simulink model "Ford_T3T6_ArchCnctnDigrm"  (R2016b)
settings: Solver=FixedStepDiscrete  StartTime=0.0  StopTime=10.0  RelTol=1e-3  EnableMultiTasking=on
libraries: canmsglib x15
(part 4 of 15)

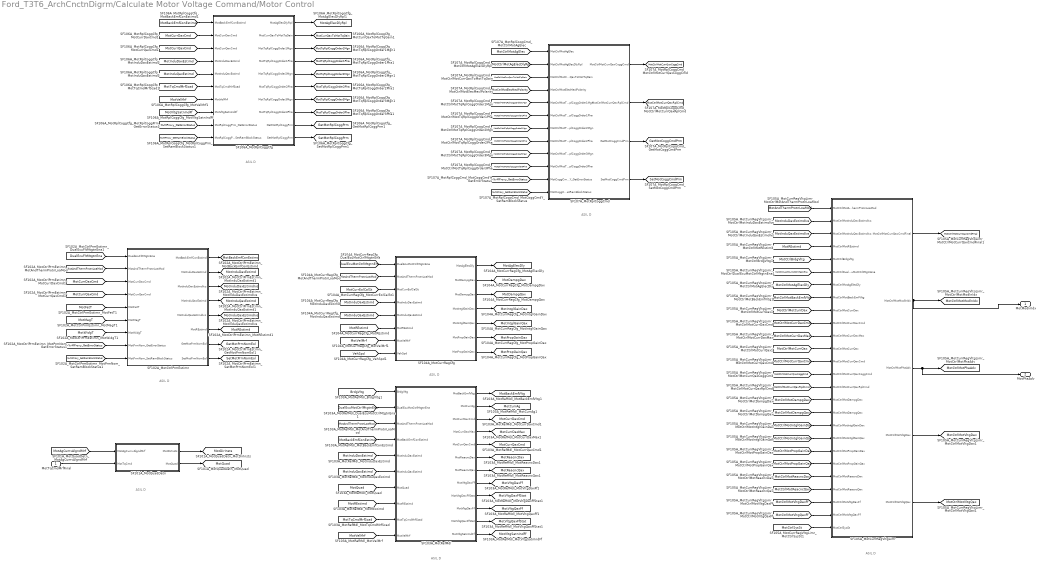
== system Ford_T3T6_ArchCnctnDigrm/Calculate Motor Voltage Command/Motor Control ==
  note: ASIL D
  note: ASIL D
  note: ASIL D
  note: ASIL D
  note: ASIL D
  note: ASIL D
  note: ASIL D
  MotTqCmdMrfFinal : Inport
  SF101A_MotQuadDetn : Subsystem  Tag=1.2.1  Description=The Motor Quadrant Detection function generates an estimate of the motor operating quadrant based on the sign of the Limited Motor Torque Command and the direction of motor shaft motion.
      settings: AttributesFormatString=Version: %<Tag>
  SF102A_MotCtrlPrmEstimn : Subsystem  Tag=3.0.0  Description=The Parameter Compensation function generates four parameter estimates: the Resistance estimate (representing the total motor output circuit resistance), the Ke estimate (representing the motor voltage constant Ke), the q-axis Motor Inductance Estimate and the d-axis Motor Inductance Estimate. The Parameter Compensation function is implemented as a feedforward parameter estimation function based on component nominal values, temperature estimates, the Motor Current Reference (q-axis and d-axis components). The temperature dependent portion of the feedforward parameter estimation function updates synchronously at the same rate as the fastest temperature estimate for the parameter (defined in the Temperature Estimation FDD).
      settings: AttributesFormatString=Version: %<Tag>
  SF103A_MotRefMdl : Subsystem  Tag=4.1.0  Description="The Motor Reference Model Function primary purpose is to calculate the reference motor current in the d/q coordinate frame to be used as the current command for the SF-104A, SF105A Current Regulator.  In general, this calculation produces the optimal (lowest) motor current command reference to produce the Motor Torque Command at the present operating point (motor velocity, supply voltage).  Features are included to use something short of the optimal reference for multiple purposes, such as to reserve some supply voltage budget for downstream current regulator operation, or for cogging/ripple cancellation, or to smooth the transition of low values of Id to high values of Id as the motor operating conditions change.  Supplementary functions include the calculation of a Feedforward Reference Voltage for use in the SF-105A Current Regulator, whose form changes depending on the state of the signal LoA State (this allows operation in Voltage Mode Control in certain fail operational states).  Another supplementary function computes the Motor Reference Current angle (Alpha) for use in the Current Measurement function."
      settings: AttributesFormatString=Version: %<Tag>
  SF104A_MotCurrRegCfg : Subsystem  Tag=3.0.0  Description=The Current Regulator Configuration function generates the following: Proportional and Integral gains for D-axis and Q-axis current regulators, damping terms for D-axis and Q-axis current regulators and a commutation delay compensation value.
      settings: AttributesFormatString=Version: %<Tag>
  SF105A_MotCurrRegVltgLimr : Subsystem  Tag=3.0.0  Description="The Current Regulator and Voltage Limiting function generates the following: Modulation Index, Phase Advance, Final Motor Current Reference Q-axis, Voltage Command D-axis and Voltage Command Q-axis.The Current Regulator portion calculates error signals representing the difference between Motor Reference Currents and Motor Measured Currents, sums in the requested motor current command from the Cogging and Ripple Command Generation function, and uses these corrected error signals modified by proportional and integral gains to generate a portion of the voltage command to the motor.  The Current Regulator also applies separate gains to the measured motor currents to generate an additional portion of the voltage command.  The Feedforward Voltages from the Motor Reference model are added to the other two portions to generate the total requested motor voltage command.The Voltage Limiting portion of the function compares the total requested motor voltage command to the total voltage available at the inverter, and implements a limiting and reference command correcting function in order to prevent windup of Current Regulator states and improve reference command tracking."
      settings: AttributesFormatString=Version: %<Tag>
  SF106A_MotRplCoggCfg : Subsystem  Tag=2.0.0  Description=This function is responsible for computing the magnitude and phase of the torque ripple and cogging torque orders to be cancelled, including base cogging and ripple values and compensation terms for the correcting for the limited bandwidth of the current regulator.
      settings: AttributesFormatString=Version: %<Tag>
  SF107A_MotRplCoggCmd : Subsystem  Tag=1.4.1  Description=This function is responsible for creating the q-axis current command for cogging and torque ripple cancellation.It runs under the time step of MotorControl x2.
      settings: AttributesFormatString=Version: %<Tag>
  MotModlnIdx : Outport
  MotPhaAdv : Outport  Port=2
  tag scope: GetMotCoggCmdPrm=global, GetMotPrmNomEol=global, GetMotRplCoggPrm=global, MotAgElecDly=global, MotAgElecDlyRpl=global, MotBackEmfConEstimd=global, MotBackEmfVltg=global, MotCtrlMotCurrQaxCmdFinal=global, MotCtrlMotCurrQaxCoggCmd=global, MotCtrlMotCurrQaxRplCmd=global, MotCtrlMotModlnIdx=global, MotCtrlMotPhaAdv=global, MotCtrlMotVltgDax=global, MotCtrlMotVltgQax=global, MotCurrAg=global, MotCurrDaxCmd=global, MotCurrDaxMax=global, MotCurrQaxCmd=global, MotCurrQaxToMotTqGain=global, MotDampgDax=global, MotDampgQax=global, MotDirInsts=global, MotInduDaxEstimd=global, MotInduDaxEstimdIvs=global, MotInduQaxEstimd=global, MotInduQaxEstimdIvs=global, MotIntglGainDax=global, MotIntglGainQax=global, MotPropGainDax=global, MotPropGainQax=global, MotQuad=global, MotREstimd=global, MotReacncDax=global, MotReacncQax=global, MotTqRplCoggOrder1Mgn=global, MotTqRplCoggOrder1Pha=global, MotTqRplCoggOrder2Mgn=global, MotTqRplCoggOrder2Pha=global, MotTqRplCoggOrder3Mgn=global, MotTqRplCoggOrder3Pha=global, MotVltgDaxFf=global, MotVltgDaxFfStat=global, MotVltgQaxFf=global, MotVltgQaxFfStat=global, MotVltgSatnIndFf=global, SetMotCoggCmdPrm=global, SetMotPrmNomEol=global, SetMotRplCoggPrm=global
  wires:
  [MotAgCumvAlgndMrf] -> SF101A_MotQuadDetn/1(MotAgCumvAlgndMrf)
  SF101A_MotQuadDetn/2(MotQuad) -> [MotQuad]
  MotTqCmdMrfFinal/1 -> SF101A_MotQuadDetn/2(MotTqCmd)
  SF101A_MotQuadDetn/1(MotDirInsts) -> [MotDirInsts]
  [MotBackEmfConEstimd] -> SF106A_MotRplCoggCfg/1(MotBackEmfConEstimd)
  [MotCurrDaxCmd] -> SF106A_MotRplCoggCfg/2(MotCurrDaxCmd)
  [MotCurrQaxCmd] -> SF106A_MotRplCoggCfg/3(MotCurrQaxCmd)
  [MotInduDaxEstimd] -> SF106A_MotRplCoggCfg/4(MotInduDaxEstimd)
  [MotInduQaxEstimd] -> SF106A_MotRplCoggCfg/5(MotInduQaxEstimd)
  [MotTqCmdMrfScad] -> SF106A_MotRplCoggCfg/6(MotTqCmdMrfScad)
  [MotVelMrf] -> SF106A_MotRplCoggCfg/7(MotVelMrf)
  [MotVltgSatnIndFf] -> SF106A_MotRplCoggCfg/8(MotVltgSatnIndFf)
  [NvMProxy_GetErrorStatus] -> SF106A_MotRplCoggCfg/9(MotRplCoggPrm_GetErrorStatus)
  [NvMProxy_SetRamBlockStatus] -> SF106A_MotRplCoggCfg/10(MotRplCoggPrm_SetRamBlockStatus)
  SF106A_MotRplCoggCfg/1(MotAgElecDlyRpl) -> [MotAgElecDlyRpl]
  SF106A_MotRplCoggCfg/2(MotCurrQaxToMotTqGain) -> [MotCurrQaxToMotTqGain]
  SF106A_MotRplCoggCfg/3(MotTqRplCoggOrder1Mgn) -> [MotTqRplCoggOrder1Mgn]
  SF106A_MotRplCoggCfg/4(MotTqRplCoggOrder1Pha) -> [MotTqRplCoggOrder1Pha]
  SF106A_MotRplCoggCfg/5(MotTqRplCoggOrder2Mgn) -> [MotTqRplCoggOrder2Mgn]
  SF106A_MotRplCoggCfg/6(MotTqRplCoggOrder2Pha) -> [MotTqRplCoggOrder2Pha]
  SF106A_MotRplCoggCfg/7(MotTqRplCoggOrder3Mgn) -> [MotTqRplCoggOrder3Mgn]
  SF106A_MotRplCoggCfg/8(MotTqRplCoggOrder3Pha) -> [MotTqRplCoggOrder3Pha]
  SF106A_MotRplCoggCfg/9(GetMotRplCoggPrm) -> [GetMotRplCoggPrm]
  SF106A_MotRplCoggCfg/10(SetMotRplCoggPrm) -> [SetMotRplCoggPrm]
  [MotAndThermProtnLoaMod] -> SF105A_MotCurrRegVltgLimr/1(MotCtrlMotAndThermProtnLoaMod)
  [MotInduDaxEstimdIvs] -> SF105A_MotCurrRegVltgLimr/2(MotCtrlMotInduDaxEstimdIvs)
  [MotInduQaxEstimdIvs] -> SF105A_MotCurrRegVltgLimr/3(MotCtrlMotInduQaxEstimdIvs)
  [MotREstimd] -> SF105A_MotCurrRegVltgLimr/4(MotCtrlMotREstimd)
  [MotCtrlBrdgVltg] -> SF105A_MotCurrRegVltgLimr/5(MotCtrlBrdgVltg)
  [MotCtrlDualEcuMotCtrlMtgtnEna] -> SF105A_MotCurrRegVltgLimr/6(MotCtrlDualEcuMotCtrlMtgtnEna)
  [MotCtrlMotAgElecDly] -> SF105A_MotCurrRegVltgLimr/7(MotCtrlMotAgElecDly)
  [MotCtrlMotBackEmfVltg] -> SF105A_MotCurrRegVltgLimr/8(MotCtrlMotBackEmfVltg)
  [MotCtrlMotCurrDax] -> SF105A_MotCurrRegVltgLimr/9(MotCtrlMotCurrDax)
  [MotCtrlMotCurrDaxCmd] -> SF105A_MotCurrRegVltgLimr/10(MotCtrlMotCurrDaxCmd)
  [MotCtrlMotCurrDaxMax] -> SF105A_MotCurrRegVltgLimr/11(MotCtrlMotCurrDaxMax)
  [MotCtrlMotCurrQax] -> SF105A_MotCurrRegVltgLimr/12(MotCtrlMotCurrQax)
  [MotCtrlMotCurrQaxCmd] -> SF105A_MotCurrRegVltgLimr/13(MotCtrlMotCurrQaxCmd)
  [MotCtrlMotCurrQaxCoggCmd] -> SF105A_MotCurrRegVltgLimr/14(MotCtrlMotCurrQaxCoggCmd)
  [MotCtrlMotCurrQaxRplCmd] -> SF105A_MotCurrRegVltgLimr/15(MotCtrlMotCurrQaxRplCmd)
  [MotCtrlMotDampgDax] -> SF105A_MotCurrRegVltgLimr/16(MotCtrlMotDampgDax)
  [MotCtrlMotDampgQax] -> SF105A_MotCurrRegVltgLimr/17(MotCtrlMotDampgQax)
  [MotCtrlMotIntglGainDax] -> SF105A_MotCurrRegVltgLimr/18(MotCtrlMotIntglGainDax)
  [MotCtrlMotIntglGainQax] -> SF105A_MotCurrRegVltgLimr/19(MotCtrlMotIntglGainQax)
  [MotCtrlMotPropGainDax] -> SF105A_MotCurrRegVltgLimr/20(MotCtrlMotPropGainDax)
  [MotCtrlMotPropGainQax] -> SF105A_MotCurrRegVltgLimr/21(MotCtrlMotPropGainQax)
  [MotCtrlMotReacncDax] -> SF105A_MotCurrRegVltgLimr/22(MotCtrlMotReacncDax)
  [MotCtrlMotReacncQax] -> SF105A_MotCurrRegVltgLimr/23(MotCtrlMotReacncQax)
  [MotCtrlMotVltgDaxFf] -> SF105A_MotCurrRegVltgLimr/24(MotCtrlMotVltgDaxFf)
  [MotCtrlMotVltgQaxFf] -> SF105A_MotCurrRegVltgLimr/25(MotCtrlMotVltgQaxFf)
  [MotCtrlSysSt] -> SF105A_MotCurrRegVltgLimr/26(MotCtrlSysSt)
  SF105A_MotCurrRegVltgLimr/1(MotCtrlMotCurrQaxCmdFinal) -> [MotCtrlMotCurrQaxCmdFinal]
  SF105A_MotCurrRegVltgLimr/2(MotCtrlMotModlnIdx) -> MotModlnIdx/1, [MotCtrlMotModlnIdx]
  SF105A_MotCurrRegVltgLimr/3(MotCtrlMotPhaAdv) -> MotPhaAdv/1, [MotCtrlMotPhaAdv]
  SF105A_MotCurrRegVltgLimr/4(MotCtrlMotVltgDax) -> [MotCtrlMotVltgDax]
  SF105A_MotCurrRegVltgLimr/5(MotCtrlMotVltgQax) -> [MotCtrlMotVltgQax]
  [DualEcuMotCtrlMtgtnEna] -> SF104A_MotCurrRegCfg/1(DualEcuMotCtrlMtgtnEna)
  [MotAndThermProtnLoaMod] -> SF104A_MotCurrRegCfg/2(MotAndThermProtnLoaMod)
  [MotCurrEolCalSt] -> SF104A_MotCurrRegCfg/3(MotCurrEolCalSt)
  [MotInduDaxEstimd] -> SF104A_MotCurrRegCfg/4(MotInduDaxEstimd)
  [MotInduQaxEstimd] -> SF104A_MotCurrRegCfg/5(MotInduQaxEstimd)
  [MotREstimd] -> SF104A_MotCurrRegCfg/6(MotREstimd)
  [MotVelMrf] -> SF104A_MotCurrRegCfg/7(MotVelMrf)
  [VehSpd] -> SF104A_MotCurrRegCfg/8(VehSpd)
  SF104A_MotCurrRegCfg/1(MotAgElecDly) -> [MotAgElecDly]
  SF104A_MotCurrRegCfg/2(MotDampgDax) -> [MotDampgDax]
  SF104A_MotCurrRegCfg/3(MotDampgQax) -> [MotDampgQax]
  SF104A_MotCurrRegCfg/4(MotIntglGainDax) -> [MotIntglGainDax]
  SF104A_MotCurrRegCfg/5(MotIntglGainQax) -> [MotIntglGainQax]
  SF104A_MotCurrRegCfg/6(MotPropGainDax) -> [MotPropGainDax]
  SF104A_MotCurrRegCfg/7(MotPropGainQax) -> [MotPropGainQax]
  [BrdgVltg] -> SF103A_MotRefMdl/1(BrdgVltg)
  [DualEcuMotCtrlMtgtnEna] -> SF103A_MotRefMdl/2(DualEcuMotCtrlMtgtnEna)
  [MotAndThermProtnLoaMod] -> SF103A_MotRefMdl/3(MotAndThermProtnLoaMod)
  [MotBackEmfConEstimd] -> SF103A_MotRefMdl/4(MotBackEmfConEstimd)
  [MotInduDaxEstimd] -> SF103A_MotRefMdl/5(MotInduDaxEstimd)
  [MotInduQaxEstimd] -> SF103A_MotRefMdl/6(MotInduQaxEstimd)
  [MotQuad] -> SF103A_MotRefMdl/7(MotQuad)
  [MotREstimd] -> SF103A_MotRefMdl/8(MotREstimd)
  [MotTqCmdMrfScad] -> SF103A_MotRefMdl/9(MotTqCmdMrfScad)
  [MotVelMrf] -> SF103A_MotRefMdl/10(MotVelMrf)
  SF103A_MotRefMdl/1(MotBackEmfVltg) -> [MotBackEmfVltg]
  SF103A_MotRefMdl/2(MotCurrAg) -> [MotCurrAg]
  SF103A_MotRefMdl/3(MotCurrDaxCmd) -> [MotCurrDaxCmd]
  SF103A_MotRefMdl/4(MotCurrDaxMax) -> [MotCurrDaxMax]
  SF103A_MotRefMdl/5(MotCurrQaxCmd) -> [MotCurrQaxCmd]
  SF103A_MotRefMdl/6(MotReacncDax) -> [MotReacncDax]
  SF103A_MotRefMdl/7(MotReacncQax) -> [MotReacncQax]
  SF103A_MotRefMdl/8(MotVltgDaxFf) -> [MotVltgDaxFf]
  SF103A_MotRefMdl/9(MotVltgDaxFfStat) -> [MotVltgDaxFfStat]
  SF103A_MotRefMdl/10(MotVltgQaxFf) -> [MotVltgQaxFf]
  SF103A_MotRefMdl/11(MotVltgQaxFfStat) -> [MotVltgQaxFfStat]
  SF103A_MotRefMdl/12(MotVltgSatnIndFf) -> [MotVltgSatnIndFf]
  [DualEcuFltMtgtnEna] -> SF102A_MotCtrlPrmEstimn/1(DualEcuFltMtgtnEna)
  [MotAndThermProtnLoaMod] -> SF102A_MotCtrlPrmEstimn/2(MotAndThermProtnLoaMod)
  [MotCurrDaxCmd] -> SF102A_MotCtrlPrmEstimn/3(MotCurrDaxCmd)
  [MotCurrQaxCmd] -> SF102A_MotCtrlPrmEstimn/4(MotCurrQaxCmd)
  [MotFetT] -> SF102A_MotCtrlPrmEstimn/5(MotFetT)
  [MotMagT] -> SF102A_MotCtrlPrmEstimn/6(MotMagT)
  [MotWidgT] -> SF102A_MotCtrlPrmEstimn/7(MotWidgT)
  [NvMProxy_GetErrorStatus] -> SF102A_MotCtrlPrmEstimn/8(MotPrmNom_GetErrorStatus)
  [NvMProxy_SetRamBlockStatus] -> SF102A_MotCtrlPrmEstimn/9(MotPrmNom_SetRamBlockStatus)
  SF102A_MotCtrlPrmEstimn/1(MotBackEmfConEstimd) -> [MotBackEmfConEstimd]
  SF102A_MotCtrlPrmEstimn/2(MotInduDaxEstimd) -> [MotInduDaxEstimd]
  SF102A_MotCtrlPrmEstimn/3(MotInduDaxEstimdIvs) -> [MotInduDaxEstimdIvs]
  SF102A_MotCtrlPrmEstimn/4(MotInduQaxEstimd) -> [MotInduQaxEstimd]
  SF102A_MotCtrlPrmEstimn/5(MotInduQaxEstimdIvs) -> [MotInduQaxEstimdIvs]
  SF102A_MotCtrlPrmEstimn/6(MotREstimd) -> [MotREstimd]
  SF102A_MotCtrlPrmEstimn/7(GetMotPrmNomEol) -> [GetMotPrmNomEol]
  SF102A_MotCtrlPrmEstimn/8(SetMotPrmNomEol) -> [SetMotPrmNomEol]
  [MotCtrlMotAgElec] -> SF107A_MotRplCoggCmd/1(MotCtrlMotAgElec)
  [MotCtrlMotAgElecDlyRpl] -> SF107A_MotRplCoggCmd/2(MotCtrlMotAgElecDlyRpl)
  [MotCtrlMotCurrQaxToMotTqGain] -> SF107A_MotRplCoggCmd/3(MotCtrlMotCurrQaxToMotTqGain)
  [MotCtrlMotElecMeclPolarity] -> SF107A_MotRplCoggCmd/4(MotCtrlMotElecMeclPolarity)
  [MotCtrlMotTqRplCoggOrder1Mgn] -> SF107A_MotRplCoggCmd/5(MotCtrlMotTqRplCoggOrder1Mgn)
  [MotCtrlMotTqRplCoggOrder1Pha] -> SF107A_MotRplCoggCmd/6(MotCtrlMotTqRplCoggOrder1Pha)
  [MotCtrlMotTqRplCoggOrder2Mgn] -> SF107A_MotRplCoggCmd/7(MotCtrlMotTqRplCoggOrder2Mgn)
  [MotCtrlMotTqRplCoggOrder2Pha] -> SF107A_MotRplCoggCmd/8(MotCtrlMotTqRplCoggOrder2Pha)
  [MotCtrlMotTqRplCoggOrder3Mgn] -> SF107A_MotRplCoggCmd/9(MotCtrlMotTqRplCoggOrder3Mgn)
  [MotCtrlMotTqRplCoggOrder3Pha] -> SF107A_MotRplCoggCmd/10(MotCtrlMotTqRplCoggOrder3Pha)
  [NvMProxy_GetErrorStatus] -> SF107A_MotRplCoggCmd/11(MotCoggCmdY_GetErrorStatus)
  [NvMProxy_SetRamBlockStatus] -> SF107A_MotRplCoggCmd/12(MotCoggCmdY_SetRamBlockStatus)
  SF107A_MotRplCoggCmd/1(MotCtrlMotCurrQaxCoggCmd) -> [MotCtrlMotCurrQaxCoggCmd]
  SF107A_MotRplCoggCmd/2(MotCtrlMotCurrQaxRplCmd) -> [MotCtrlMotCurrQaxRplCmd]
  SF107A_MotRplCoggCmd/3(GetMotCoggCmdPrm) -> [GetMotCoggCmdPrm]
  SF107A_MotRplCoggCmd/4(SetMotCoggCmdPrm) -> [SetMotCoggCmdPrm]

== system Ford_T3T6_ArchCnctnDigrm/Calculate Motor Voltage Command/SF019B_PwrLimr ==
  AltFltActv : Inport
  BrdgVltg : Inport  Port=2
  DualEcuFltMtgtnSca : Inport  Port=3
  MotAndThermProtnLoaMod : Inport  Port=4
  MotBackEmfConEstimd : Inport  Port=5
  MotTqCmdMrf : Inport  Port=6
  MotVelMrf : Inport  Port=7
  GetRefTmr100MicroSec32bit : Inport  Port=8
  GetTiSpan100MicroSec32bit : Inport  Port=9
  SetNtcSts : Inport  Port=10
  MotTqCmdPwrLimd : Outport
  PwrLimrRednFac : Outport  Port=2

== system Ford_T3T6_ArchCnctnDigrm/Calculate Motor Voltage Command/SF032A_MotTqCmdSca1 ==
  MotTqCmdMrf : Inport
  MotTqScaFac_GetErrorStatus : Inport  Port=2
  MotTqScaFac_SetRamBlockStatus : Inport  Port=3
  MotTqCmdMrfScad : Outport
  GetMotTqCmdSca : Outport  Port=2
  SetMotTqCmdSca : Outport  Port=3

== system Ford_T3T6_ArchCnctnDigrm/Calculate Motor Voltage Command/SF050A_MotTqTranlDampg ==
  AssiMechPolarity : Inport
  DiagcStsCtrldShtDwnFltPrsnt : Inport  Port=2
  HwAg : Inport  Port=3
  LoaSt : Inport  Port=4
  MotTqCmdCrf : Inport  Port=5
  MotVelCrf : Inport  Port=6
  SysSt : Inport  Port=7
  VehSpd : Inport  Port=8
  GetRefTmr100MicroSec32bit : Inport  Port=9
  GetTiSpan100MicroSec32bit : Inport  Port=10
  MotTqCmdCrfDampd : Outport
  MotTqCmdMrfDampd : Outport  Port=2
  MotTqTranlDampgCmpl : Outport  Port=3

== system Ford_T3T6_ArchCnctnDigrm/Complex Drivers/AR102B_NxtrTi ==
  ClrErrInjReg : Inport
  ReadErrInjReg : Inport  Port=2
  SetNtcSts : Inport  Port=3
  GetRefTmr100MicroSec32bit : Outport
  GetRefTmr1MicroSec32bit : Outport  Port=2
  GetTiSpan100MicroSec32bit : Outport  Port=3
  GetTiSpan1MicroSec32bit : Outport  Port=4

== system Ford_T3T6_ArchCnctnDigrm/Complex Drivers/CM101B_ExcpnHndlg ==
  SetNtcSts : Inport
  SetNtcStsAndSnpshtData : Inport  Port=2
  ChkForStrtUpTest : Outport
  FeNmiBusBrdgErr : Outport  Port=2
  FeNmiBusSngBitEccErr : Outport  Port=3
  FeNmiClkMonr0RtErr : Outport  Port=4
  FeNmiClkMonr1RtErr : Outport  Port=5
  FeNmiClkMonr2RtErr : Outport  Port=6
  FeNmiClkMonr3RtErr : Outport  Port=7
  FeNmiClkMonr5RtErr : Outport  Port=8
  FeNmiCodFlsEccAdrOvfErr : Outport  Port=9
  FeNmiCodFlsIllglAcsBySysBus : Outport  Port=10
  FeNmiDmaIllglAcsErr : Outport  Port=11
  FeNmiDmaLockStepErrOrGblRamWrBufErr : Outport  Port=12
  FeNmiDmaTrfErr : Outport  Port=13
  FeNmiDtsRamDblBitEccErr : Outport  Port=14
  FeNmiEcmMstChkrErr : Outport  Port=15
  FeNmiFlsSeqErr : Outport  Port=16
  FeNmiGblRamIllglAcsByProcr : Outport  Port=17
  FeNmiGblRamIllglAcsBySysBus : Outport  Port=18
  FeNmiGlbRamEccAdrOvfErr : Outport  Port=19
  FeNmiGtmRamDblBitEccErr : Outport  Port=20
  FeNmiLclRamEccAdrOvfErr : Outport  Port=21
  FeNmiModErrDbgActv : Outport  Port=22
  FeNmiModErrProgmModActv : Outport  Port=23
  FeNmiModErrTestModActv : Outport  Port=24
  FeNmiModErrUsrModInactv : Outport  Port=25
  FeNmiPegErr : Outport  Port=26
  FeNmiProcrLockStepErr : Outport  Port=27
  FeNmiPrphlRamEccAdrOvfErr : Outport  Port=28
  FeNmiResdAreaIllglAcsByHiSpdBus : Outport  Port=29
  FeNmiWdgErr : Outport  Port=30
  GetMcuDiagcIdnData : Outport  Port=31
  GetMcuDiagcSpplData : Outport  Port=32
  ProcMpuExcpnErr : Outport  Port=33
  ProcNonCritOsErr : Outport  Port=34
  ProcPrmntOsErr : Outport  Port=35
  ProcPrvlgdInstrExcpnErr : Outport  Port=36
  ProcUkwnExcpnErr : Outport  Port=37
  SetMcuDiagcIdnData : Outport  Port=38

== system Ford_T3T6_ArchCnctnDigrm/Complex Drivers/CM102B_FlsMem ==
  ChkForStrtUpTest : Inport
  GetRefTmr100MicroSec32bit : Inport  Port=2
  GetTiSpan100MicroSec32bit : Inport  Port=3
  ResvCrcHwUnit : Inport  Port=4
  SetNtcSts : Inport  Port=5
  CodFlsCrcChkCmpl : Outport
  SwApplCrc : Outport  Port=2

== system Ford_T3T6_ArchCnctnDigrm/Complex Drivers/CM103B_RamMem ==
  SetNtcSts : Inport
  GlbRamEccSngBitCntrOutp : Outport
  LclRamEccSngBitCntrOutp : Outport  Port=2

== system Ford_T3T6_ArchCnctnDigrm/Complex Drivers/CM104B_EcmOutpAndDiagc ==
  ChkForStrtUpTest : Inport
  GetMcuDiagcIdnData : Inport  Port=2
  SetMcuDiagcIdnData : Inport  Port=3
  CtrlErrOut : Outport

== system Ford_T3T6_ArchCnctnDigrm/Complex Drivers/CM106B_McuCoreCfgAndDiagc ==
  GetMcuDiagcIdnData : Inport
  SetMcuDiagcIdnData : Inport  Port=2

== system Ford_T3T6_ArchCnctnDigrm/Complex Drivers/CM109B_ClkCfgAndMon ==

== system Ford_T3T6_ArchCnctnDigrm/Complex Drivers/CM800A_SyncCrc ==
  Calc16BitCrc_u08 : Outport
  Calc16BitCrc_u16 : Outport  Port=2
  Calc32BitCrc_u08 : Outport  Port=3
  Calc32BitCrc_u16 : Outport  Port=4
  Calc32BitCrc_u32 : Outport  Port=5
  Calc8BitCrc : Outport  Port=6
  Calc8BitCrc0X2F : Outport  Port=7
  ResvCrcHwUnit : Outport  Port=8

== system Ford_T3T6_ArchCnctnDigrm/Complex Drivers/ES104B_XcpIf ==

== system Ford_T3T6_ArchCnctnDigrm/Complex Drivers/Ford001A_ChkPt ==

== system Ford_T3T6_ArchCnctnDigrm/Complex Drivers/Platform Config ==
  note: how to connect to fast loop??
  note: Not Required
      | Using only one HwAg Sensor
  note: Not Required
      | Using only 4 HwTq Sensors
  note: Not Required
      | Using only 3 MotAg Sensors
  note: how to connect to fast loop??
  note: how to connect to fast loop??
  note: ASIL D
  note: ASIL D
  note: ASIL D
  note: ASIL D
  CM107B_GuardCfgAndDiagc : Subsystem  Tag=1.2.0  Description=FDD that contians guard configuration for PEG, IPG, HBG, GRG and PBG
      settings: AttributesFormatString=Version: %<Tag>
  CM201A_DmaCfgAndUse : Subsystem  Tag=1.2.0  Description=DMA Configuration and Usage
      settings: AttributesFormatString=Version: %<Tag>
  CM301A_Adcf0CfgAndUse : Subsystem  Tag=1.1.0  Description="This FDD is responsible for configuring and use of the Adcf0.  This is the Adc sampled at the motor control rate."
      settings: AttributesFormatString=Version: %<Tag>
  CM321A_Adcf1CfgAndUse : Subsystem  Tag=1.1.0  Description="This FDD is responsible for configuring and use of the ADC1.  This is the ADC sampled at the 2mSec rate."
      settings: AttributesFormatString=Version: %<Tag>
  ES102A_PolarityCfg : Subsystem  Tag=1.4.0  Description=Identifies polarity control settings for certain points in the design
      settings: AttributesFormatString=Version: %<Tag>
  tag scope: Adcf1EnaCnvn=global, AssiMechPolarity=global, DmaEna2MilliSecToMotCtrlTrf=global, DmaWaitForMotCtrlTo2MilliSecTrf=global, HwAgAPolarity=global, HwAgBPolarity=global, HwAgCPolarity=global, HwAgDPolarity=global, HwAgEPolarity=global, HwAgFPolarity=global, HwAgGPolarity=global, HwAgHPolarity=global, HwTqAPolarity=global, HwTqBPolarity=global, HwTqCPolarity=global, HwTqDPolarity=global, HwTqEPolarity=global, HwTqFPolarity=global, HwTqGPolarity=global, HwTqHPolarity=global, InjDmaErr=global, InjMcuDiagcErr=global, MotAgMeclAPolarity=global, MotAgMeclBPolarity=global, MotAgMeclCPolarity=global, MotAgMeclDPolarity=global, MotAgMeclEPolarity=global, MotAgMeclFPolarity=global, MotAgMeclGPolarity=global, MotAgMeclHPolarity=global, MotCtrlAdc0RawRes=global, MotCtrlAdc1RawRes=global, MotCtrlMgr_MotCtrlFromTwoMilliSec_Rec=global, MotCtrlMgr_TwoMilliSecFromMotCtrl_Rec=global, MotElecMeclPolarity=global, PolarityCfgRead=global, PolarityCfgWr=global
  wires:
  [MotCtrlAdcDiagcEndPtrOutp] -> CM301A_Adcf0CfgAndUse/1(MotCtrlAdcDiagcEndPtrOutp)
  [MotCtrlAdcDiagcStrtPtrOutp] -> CM301A_Adcf0CfgAndUse/2(MotCtrlAdcDiagcStrtPtrOutp)
  [AdcDiagcEndPtrOutp] -> CM321A_Adcf1CfgAndUse/1(AdcDiagcEndPtrOutp)
  [AdcDiagcStrtPtrOutp] -> CM321A_Adcf1CfgAndUse/2(AdcDiagcStrtPtrOutp)
  CM321A_Adcf1CfgAndUse/1(Adcf1EnaCnvn) -> [Adcf1EnaCnvn]
  [MotCtrlMgr_MotCtrlToTwoMilliSec_Rec] -> CM201A_DmaCfgAndUse/1(MotCtrlMgr_MotCtrlToTwoMilliSec_Rec)
  [MotCtrlMgr_TwoMilliSecToMotCtrl_Rec] -> CM201A_DmaCfgAndUse/2(MotCtrlMgr_TwoMilliSecToMotCtrl_Rec)
  [Adc1CfgAndUseAdc1EnaCnvn] -> CM201A_DmaCfgAndUse/3(Adc1CfgAndUseAdc1EnaCnvn)
  [ClrErrInjReg] -> CM201A_DmaCfgAndUse/4(ClrErrInjReg)
  [GetRefTmr1MicroSec32bit] -> CM201A_DmaCfgAndUse/5(GetRefTmr1MicroSec32bit)
  [GetTiSpan1MicroSec32bit] -> CM201A_DmaCfgAndUse/6(GetTiSpan1MicroSec32bit)
  [ReadErrInjReg] -> CM201A_DmaCfgAndUse/7(ReadErrInjReg)
  [StrtErrInjCntr] -> CM201A_DmaCfgAndUse/8(StrtErrInjCntr)
  CM201A_DmaCfgAndUse/1(MotCtrlAdc0RawRes) -> [MotCtrlAdc0RawRes]
  CM201A_DmaCfgAndUse/2(MotCtrlAdc1RawRes) -> [MotCtrlAdc1RawRes]
  CM201A_DmaCfgAndUse/3(MotCtrlMgr_MotCtrlFromTwoMilliSec_Rec) -> [MotCtrlMgr_MotCtrlFromTwoMilliSec_Rec]
  CM201A_DmaCfgAndUse/4(MotCtrlMgr_TwoMilliSecFromMotCtrl_Rec) -> [MotCtrlMgr_TwoMilliSecFromMotCtrl_Rec]
  CM201A_DmaCfgAndUse/5(DmaEna2MilliSecToMotCtrlTrf) -> [DmaEna2MilliSecToMotCtrlTrf]
  CM201A_DmaCfgAndUse/6(DmaWaitForMotCtrlTo2MilliSecTrf) -> [DmaWaitForMotCtrlTo2MilliSecTrf]
  CM201A_DmaCfgAndUse/7(InjDmaErr) -> [InjDmaErr]
  CM201A_DmaCfgAndUse/8(InjMcuDiagcErr) -> [InjMcuDiagcErr]
  [NvMProxy_SetRamBlockStatus] -> ES102A_PolarityCfg/1(PolarityCfgSaved_SetRamBlockStatus)
  ES102A_PolarityCfg/1(AssiMechPolarity) -> [AssiMechPolarity]
  ES102A_PolarityCfg/2(HwAgAPolarity) -> [HwAgAPolarity]
  ES102A_PolarityCfg/3(HwAgBPolarity) -> [HwAgBPolarity]
  ES102A_PolarityCfg/4(HwAgCPolarity) -> [HwAgCPolarity]
  ES102A_PolarityCfg/5(HwAgDPolarity) -> [HwAgDPolarity]
  ES102A_PolarityCfg/6(HwAgEPolarity) -> [HwAgEPolarity]
  ES102A_PolarityCfg/7(HwAgFPolarity) -> [HwAgFPolarity]
  ES102A_PolarityCfg/8(HwAgGPolarity) -> [HwAgGPolarity]
  ES102A_PolarityCfg/9(HwAgHPolarity) -> [HwAgHPolarity]
  ES102A_PolarityCfg/10(HwTqAPolarity) -> [HwTqAPolarity]
  ES102A_PolarityCfg/11(HwTqBPolarity) -> [HwTqBPolarity]
  ES102A_PolarityCfg/12(HwTqCPolarity) -> [HwTqCPolarity]
  ES102A_PolarityCfg/13(HwTqDPolarity) -> [HwTqDPolarity]
  ES102A_PolarityCfg/14(HwTqEPolarity) -> [HwTqEPolarity]
  ES102A_PolarityCfg/15(HwTqFPolarity) -> [HwTqFPolarity]
  ES102A_PolarityCfg/16(HwTqGPolarity) -> [HwTqGPolarity]
  ES102A_PolarityCfg/17(HwTqHPolarity) -> [HwTqHPolarity]
  ES102A_PolarityCfg/18(MotAgMeclAPolarity) -> [MotAgMeclAPolarity]
  ES102A_PolarityCfg/19(MotAgMeclBPolarity) -> [MotAgMeclBPolarity]
  ES102A_PolarityCfg/20(MotAgMeclCPolarity) -> [MotAgMeclCPolarity]
  ES102A_PolarityCfg/21(MotAgMeclDPolarity) -> [MotAgMeclDPolarity]
  ES102A_PolarityCfg/22(MotAgMeclEPolarity) -> [MotAgMeclEPolarity]
  ES102A_PolarityCfg/23(MotAgMeclFPolarity) -> [MotAgMeclFPolarity]
  ES102A_PolarityCfg/24(MotAgMeclGPolarity) -> [MotAgMeclGPolarity]
  ES102A_PolarityCfg/25(MotAgMeclHPolarity) -> [MotAgMeclHPolarity]
  ES102A_PolarityCfg/26(MotElecMeclPolarity) -> [MotElecMeclPolarity]
  ES102A_PolarityCfg/27(PolarityCfgRead) -> [PolarityCfgRead]
  ES102A_PolarityCfg/28(PolarityCfgWr) -> [PolarityCfgWr]

== system Ford_T3T6_ArchCnctnDigrm/Development/DF001A_FltInj ==
  HwVel : Inport
  GetRefTmr100MicroSec32bit : Inport  Port=2
  GetTiSpan100MicroSec32bit : Inport  Port=3
  FltInj_f32 : Outport
  FltInj_logl : Outport  Port=2
  FltInj_u08 : Outport  Port=3
  FltInj_u0p16 : Outport  Port=4

== system Ford_T3T6_ArchCnctnDigrm/Ford CFs/Customer Diag Services ==
  note: EED0
  note: DE00
  note: 3F964_REQ_05050300v2: SES
      | End of Travel Learning
      |
      | SES_Enabled (Software End Stops) Boolean
      | SESCompensatedSPA
      | EndStopsLearned
      | MaxAngleTavel
      | SESRampDownRate
      | SESDampUpRate
  note: EAC: External Angle Command: Kind of automated steering
  note: ANC_Enabled
      | No Units
      | Bool
      |
      | PDC_Enabled
      | No Units
      | Bool
      |
      | TSC_Enabled
      | No Units
      | Bool
      |
      | BPR_Enabled
      | No Units
      | Bool
      |
      | LKA_Enabled
      | No Units
      | Bool
      |
      | LDW_Enabled
      | No Units
      | Bool
      |
      | TJA_Enabled
      | No Units
      | Bool
      |
      | LCA_Enabled
      | No Units
      | Bool
      |
      | TBA_Enabled
      | No Units
      | Bool
      |
      | TBA_5_Wheel_Enabled
      | No Units
      | Bool
      |
      | TBA_TRG_Enabled
      | No Units
      | Bool
      |
      | ESA_Enabled
      | No Units
      | Bool
      |
      | DSR_Enabled
      | No Units
      | Bool
      |
      | SAPP/APA_Enabled
      | No Units
      | Bool
      |
      | SES_Enabled
      | No Units
      | Bool
      |
      | StartStop_Enabled (StrtStopDIDSt)
      | No Units
      | U-8
      |
      | ActiveReturn_Enabled
      | No Units
      | Bool
      |
      | SDM_Enabled
      | No Units
      | Bool
      |
      | RF_Enabled
      | No Units
      | Bool
      |
      | AFS_Present
      | No Units
      | Bool
  note: DE00 Byte 5
  note: DE02 Byte 1
  note: DE01 Byte 1
  note: DE00 Byte 4
  note: DE01 Byte 2
  note: DE01 Byte 3
  note: DE01 Byte 4 ??
  note: DE02 Byte 4 ??
  note: DE01 Byte 5
  note: DE01 Byte 6
  note: DE01 Byte 7
  note: DE01 Byte 8
  note: DE01 Byte 9
  note: DE01 Byte 9
  note: DE01 Byte 9
  note: DE01 Byte 10
  note: DE01 Byte 23
  note: DE02 Byte 5
  note: DE02 Byte 6
  note: DE01 Byte 5
  note: DE01
  note: DE02
  note: DE03
  note: EE00
  note: EE01
  note: EE02
  note: EE20
  note: EE21
  note: EE22
  note: EE23
  note: EE40
  note: EE41
  note: EE42
  note: EE43
  note: EE80
  note: EED1
  note: EED2
  CF086_FordDiagcSrvHndlg : Subsystem  Tag=1.0.X  Description=Ford DID Flag
      settings: AttributesFormatString=Version: %<Tag>
  CF088A_FordDualEcuFltDiagcCom : Subsystem  Tag=1.0.X  Description=The Ford Dual ECU Fault Diagnostic Communication function arbitrates NTCsbetween ECU 1 and ECU 2 and appropriately maps them to CTCs.
      settings: AttributesFormatString=Version: %<Tag>
  tag scope: ActvFrntSteerPrsnt=global, ActvRtnEnad=global, DrvrSteerRcmdnEnad=global, EngTqClass=global, ExtAgCtrlEnad=global, FordAbsPrsnt=global, FordActvNiblCtrlEnad=global, FordActvParkAssiEnad=global, FordBrkOscnRednEnad=global, FordBrkPlsRejctnEnad=global, FordDtcIdx=global, FordDtcSts=global, FordEscPrsnt=global, FordEvasSteerAssiEnad=global, FordLaneCentrAssiEnad=global, FordLaneDprtrWarnEnad=global, FordLaneKeepAssiEnad=global, FordPullDriftCmpEnad=global, FordResrchFctEnad=global, FordSelDrvModEnad=global, FordTqSteerCmpEnad=global, FordTrfcJamAssiEnad=global, FordTrlrBackupAssi5WhlEnad=global, FordTrlrBackupAssiEnad=global, FordTrlrBackupAssiTRGEnad=global, FordVehLoSpdMtnCtrlBrkDecelEna=global, FordWrSrvActvNiblCmpIntSts=global, FordWrSrvBrkPlsRednActvnCntr=global, FordWrSrvEvasSteerAssiIntSts=global, FordWrSrvFordExtAgCtrlStsInt=global, FordWrSrvLaneDprtrWarnIntSts=global, FordWrSrvLaneKeepAssiIntSts=global, FordWrSrvLatCtrlIntSts=global, FordWrSrvPullDriftCmpIntSts=global, FordWrSrvSteerTqDstbcRejctnIntSts=global, FordWrSrvTqSteerCmpActvnCntr=global, FordWrSrvTrlrBackupAssiIntSts=global, HwVrnt=global, IgnCycCntr=global, LaneDetnWarnEnad=global, LimpHomeDtcCntr=global, ProgsnCntr=global, SrvPullDriftCmpRstVal=global, StrtStopEnadSt=global, SwEndStopEnad=global, TunVrnt=global
  wires:
  CF086_FordDiagcSrvHndlg/1(WrSrvDrvrSteerRcmdnEnad) -> [DrvrSteerRcmdnEnad]
  CF086_FordDiagcSrvHndlg/2(WrSrvExtAgCtrlEnad) -> [ExtAgCtrlEnad]
  CF086_FordDiagcSrvHndlg/3(WrSrvFordAbsPrsnt) -> [FordAbsPrsnt]
  CF086_FordDiagcSrvHndlg/4(WrSrvFordActvNiblCtrlEnad) -> [FordActvNiblCtrlEnad]
  CF086_FordDiagcSrvHndlg/5(WrSrvFordWrSrvActvParkAssiEnad) -> [FordActvParkAssiEnad]
  CF086_FordDiagcSrvHndlg/6(WrSrvFordBrkOscnRednEnad) -> [FordBrkOscnRednEnad]
  CF086_FordDiagcSrvHndlg/7(WrSrvFordBrkPlsRejctnEnad) -> [FordBrkPlsRejctnEnad]
  CF086_FordDiagcSrvHndlg/8(WrSrvFordEvasSteerAssiEnad) -> [FordEvasSteerAssiEnad]
  CF086_FordDiagcSrvHndlg/9(WrSrvFordLaneCentrAssiEnad) -> [FordLaneCentrAssiEnad]
  CF086_FordDiagcSrvHndlg/10(WrSrvFordLaneDprtrWarnEnad) -> [FordLaneDprtrWarnEnad]
  CF086_FordDiagcSrvHndlg/11(WrSrvFordLaneKeepAssiEnad) -> [FordLaneKeepAssiEnad]
  CF086_FordDiagcSrvHndlg/12(WrSrvFordPullDriftCmpEnad) -> [FordPullDriftCmpEnad]
  CF086_FordDiagcSrvHndlg/13(WrSrvFordResrchFctEnad) -> [FordResrchFctEnad]
  CF086_FordDiagcSrvHndlg/14(WrSrvFordSelctvDrvModEnad) -> [FordSelDrvModEnad]
  CF086_FordDiagcSrvHndlg/15(WrSrvFordTqSteerCmpEnad) -> [FordTqSteerCmpEnad]
  CF086_FordDiagcSrvHndlg/16(WrSrvFordTrfcJamAssiEnad) -> [FordTrfcJamAssiEnad]
  CF086_FordDiagcSrvHndlg/17(WrSrvFordTrlrBackupAssi5WhlEnad) -> [FordTrlrBackupAssi5WhlEnad]
  CF086_FordDiagcSrvHndlg/18(WrSrvFordTrlrBackupAssiEnad) -> [FordTrlrBackupAssiEnad]
  CF086_FordDiagcSrvHndlg/19(WrSrvFordTrlrBackupAssiTRGEnad) -> [FordTrlrBackupAssiTRGEnad]
  CF086_FordDiagcSrvHndlg/20(WrSrvFordVehLoSpdMtnCtrlBrkDecelEna) -> [FordVehLoSpdMtnCtrlBrkDecelEna]
  CF086_FordDiagcSrvHndlg/21(WrSrvLaneDetnWarnEnad) -> [LaneDetnWarnEnad]
  CF086_FordDiagcSrvHndlg/22(WrSrvActvFrntSteerPrsnt) -> [ActvFrntSteerPrsnt]
  CF086_FordDiagcSrvHndlg/23(WrSrvStrtStopEnadSt) -> [StrtStopEnadSt]
  CF086_FordDiagcSrvHndlg/24(WrSrvActvRtnEnad) -> [ActvRtnEnad]
  CF086_FordDiagcSrvHndlg/25(WrSrvSwEndStopEnad) -> [SwEndStopEnad]
  [EcuId] -> CF088A_FordDualEcuFltDiagcCom/1(EcuId)
  [Dem_GetEventStatus] -> CF088A_FordDualEcuFltDiagcCom/2(Dem_GetEventStatus)
  [GetSigImcData_u08] -> CF088A_FordDualEcuFltDiagcCom/3(GetSigImcData_u08)
  [SetNtcSts10] -> CF088A_FordDualEcuFltDiagcCom/4(SetNtcSts)
  CF088A_FordDualEcuFltDiagcCom/1(FordDtcIdx) -> [FordDtcIdx]
  CF088A_FordDualEcuFltDiagcCom/2(FordDtcSts) -> [FordDtcSts]
  CF086_FordDiagcSrvHndlg/26(WrSrvIgnCycCntr) -> [IgnCycCntr]
  CF086_FordDiagcSrvHndlg/27(WrSrvFordEscPrsnt) -> [FordEscPrsnt]
  CF086_FordDiagcSrvHndlg/28(WrSrvLimpHomeDtcCntr) -> [LimpHomeDtcCntr]
  CF086_FordDiagcSrvHndlg/29(WrSrvProgsnCntr) -> [ProgsnCntr]
  CF086_FordDiagcSrvHndlg/30(WrSrvHwVrnt) -> [HwVrnt]
  CF086_FordDiagcSrvHndlg/31(WrSrvTunVrnt) -> [TunVrnt]
  CF086_FordDiagcSrvHndlg/32(WrSrvFordTqSteerCmpActvnCntr) -> [FordWrSrvTqSteerCmpActvnCntr]
  CF086_FordDiagcSrvHndlg/33(WrSrvFordBrkPlsRednActvnCntr) -> [FordWrSrvBrkPlsRednActvnCntr]
  CF086_FordDiagcSrvHndlg/34(WrSrvSrvPullDriftCmpRstVal) -> [SrvPullDriftCmpRstVal]
  CF086_FordDiagcSrvHndlg/35(WrSrvActvNiblCmpIntSts) -> [FordWrSrvActvNiblCmpIntSts]
  CF086_FordDiagcSrvHndlg/36(WrSrvFordLaneKeepAssiIntSts) -> [FordWrSrvLaneKeepAssiIntSts]
  CF086_FordDiagcSrvHndlg/37(WrSrvPullDriftCmpIntSts) -> [FordWrSrvPullDriftCmpIntSts]
  CF086_FordDiagcSrvHndlg/38(WrSrvFordLaneDprtrWarnIntSts) -> [FordWrSrvLaneDprtrWarnIntSts]
  CF086_FordDiagcSrvHndlg/39(WrSrvFordSteerTqDstbcRejctnIntSts) -> [FordWrSrvSteerTqDstbcRejctnIntSts]
  CF086_FordDiagcSrvHndlg/40(WrSrvFordEvasSteerAssiIntSts) -> [FordWrSrvEvasSteerAssiIntSts]
  CF086_FordDiagcSrvHndlg/41(WrSrvLatCtrlIntStsIntSts) -> [FordWrSrvLatCtrlIntSts]
  CF086_FordDiagcSrvHndlg/42(WrSrvTrlrBackupAssiIntSts) -> [FordWrSrvTrlrBackupAssiIntSts]
  CF086_FordDiagcSrvHndlg/44(WrSrvEngTqClass) -> [EngTqClass]
  CF086_FordDiagcSrvHndlg/43(WrSrvFordExtAgCtrlStsInt) -> [FordWrSrvFordExtAgCtrlStsInt]
  [FordHwVel] -> CF086_FordDiagcSrvHndlg/2(SPAVelocity)
  [FordCmpdHwPosn] -> CF086_FordDiagcSrvHndlg/3(CompensatedSPA)
  [HwTq] -> CF086_FordDiagcSrvHndlg/4(SteeringColumnTorque)
  [FordVehSteerPinionAgOffsRaw] -> CF086_FordDiagcSrvHndlg/5(StePinOffst_An_Est)
  [BrdgVltg] -> CF086_FordDiagcSrvHndlg/7(EPSVoltage)
  [EcuTFild] -> CF086_FordDiagcSrvHndlg/8(Internal Temp Used)
  [MotCtrlMotCurrQax] -> CF086_FordDiagcSrvHndlg/9(Q-axis Motor Current)
  [FordVehGlbRealTi] -> CF086_FordDiagcSrvHndlg/10(Global Real Time from HSCAN)
  [FordVehOdom] -> CF086_FordDiagcSrvHndlg/11(Total Distance from HSCAN)
  [FordVehOutdAirTRaw] -> CF086_FordDiagcSrvHndlg/12(VehSpd)
  [FordVehIdnNr] -> CF086_FordDiagcSrvHndlg/64(Vehicle Identification Number)
  [ActvNiblCmpIntSts] -> CF086_FordDiagcSrvHndlg/36(ReadSrvActvNiblCmpIntSts)
  [LaneDprtrWarnIntSts] -> CF086_FordDiagcSrvHndlg/37(ReadSrvLaneDprtrWarnIntSts)
  [LaneKeepAssiIntSts] -> CF086_FordDiagcSrvHndlg/38(ReadSrvLaneKeepAssiIntSts)
  [LatCtrlIntSts] -> CF086_FordDiagcSrvHndlg/39(ReadSrvLatCtrlIntSts)
  [PullDriftCmpIntSts] -> CF086_FordDiagcSrvHndlg/40(ReadSrvPullDriftCmpIntSts)
  [SrvPullDriftCmpAct] -> CF086_FordDiagcSrvHndlg/41(SrvPullDriftCmpAct)
  [TrlrBackupAssiIntSts] -> CF086_FordDiagcSrvHndlg/42(ReadSrvTrlrBackupAssiIntSts)
  [FordSteerTqDstbcRejctnIntSts] -> CF086_FordDiagcSrvHndlg/43(ReadSrvFordSteerTqDstbcRejctnIntSts)
  [FordEvasSteerAssiIntSts] -> CF086_FordDiagcSrvHndlg/44(ReadSrvFordEvasSteerAssiIntSts)
  [FordTqSteerCmpActvnCntr] -> CF086_FordDiagcSrvHndlg/45(ReadSrvFordTqSteerCmpActvnCntr)
  [FordBrkPlsRednActvnCntr] -> CF086_FordDiagcSrvHndlg/46(ReadSrvFordBrkPlsRednActvnCntr)
  [FordVehOutdAirT] -> CF086_FordDiagcSrvHndlg/13(FordVehOutdAirT)
  [FordVehGlbRealTi] -> CF086_FordDiagcSrvHndlg/14(FordVehGlbRealTi)
  [FordAppldFinalMotTq] -> CF086_FordDiagcSrvHndlg/24(AppliedFinalMotorTorque)

== system Ford_T3T6_ArchCnctnDigrm/Ford CFs/FIH Read and Write ==
  note: // Write --> data flow from FIH to nexteer
  note: // Read --> The Vehicle Physical Parameters (e.g. Wheelbase, Rack-to-Pinion Ratio, etc.) must be provided by Base EPS to In-House Features via Software
      | Read Functions. In-House Features that require these parameters will request it once during Initialization.
  FIH Initialize : Subsystem
  FIH Read : Subsystem
  FIH write : Subsystem
